simulink library "lib_dGrid"  (R2023b)
settings: Solver=VariableStepAuto  StartTime=0.0  StopTime=10.0  RelTol=1e-3
values from neighbouring files (symbols this model uses):
  C_PM = 10e-3    (= 0.01)    [my_MMC_param.m]
  Cbase = 1/Zbase/wb    (= 3.10849498226e-05)    [my_MMC_param.m]
  f0 = 50/fb    (= 1)    [my_MMC_param.m]
  Fn_filter = 1000    [my_MMC_param.m]
  Fnom = 50    [my_MMC_param.m]
  GFL_APC = 1    [Analysis_Main.m]    (also in initSimu.m; my_MMC_param.m)
  GFL_DVC = 2    [Analysis_Main.m]    (also in initSimu.m; my_MMC_param.m)
  GFM_APC = 3; (values programmed in EMT models)    [Analysis_Main.m]    (also in initSimu.m; my_MMC_param.m = 3)
  GFM_VF = 0    [my_MMC_param.m]
  Ibase = 2*Sbase/(3*Ubase)    [my_MMC_param.m]
  Idcb = Sbase/Udcb    [my_MMC_param.m]
  Ki_Iccsc = 5.15    [my_MMC_param.m]
  Ki_Ireg = CCCTRL.CC.ki    [my_MMC_param.m]
  Ki_Izscc = 100    [my_MMC_param.m]
  Ki_PLL = 1/(CCCTRL.PLL.v0*CCCTRL.PLL.T^2)    [my_MMC_param.m]
  Ki_Preg = 1.0*10    (= 10)    [my_MMC_param.m]
  Ki_Qreg = 1.0*10    (= 10)    [my_MMC_param.m]
  Ki_VAC_GFL = 50    [my_MMC_param.m]
  Ki_VACreg = 10    [my_MMC_param.m]
  Ki_VDCreg = 10    [my_MMC_param.m]
  Ki_WtReg = Kp_WtReg / 0.025    (= 1600)    [my_MMC_param.m]
  Kp_Iccsc = 0.21    [my_MMC_param.m]
  Kp_Ireg = CCCTRL.CC.kp    [my_MMC_param.m]
  Kp_Izscc = 10    [my_MMC_param.m]
  Kp_PLL = 2/CCCTRL.PLL.v0/CCCTRL.PLL.T    [my_MMC_param.m]
  Kp_Preg = 0.5/3*1    (= 0.166666666667)    [my_MMC_param.m]
  Kp_Qreg = 0.5/3*1    (= 0.166666666667)    [my_MMC_param.m]
  Kp_VAC_GFL = 0.5    [my_MMC_param.m]
  Kp_VACreg = 0.01    [my_MMC_param.m]
  Kp_VDCreg = 1    [my_MMC_param.m]
  Kp_WtReg = 40    [my_MMC_param.m]
  Kpv_GFM = 1    [my_MMC_param.m]
  Kpwm = 0.5    [my_MMC_param.m]
  Larm = Larm_pu*(Zbase/wb)    (= 0.0488923985178)    [my_MMC_param.m]
  Lff = Larm_pu/2    (= 0.075)    [my_MMC_param.m]
  Limits_Ireg = [ 2.0  -2.0]    [my_MMC_param.m]
  Limits_Preg = [ 2, -2 ]    [my_MMC_param.m]
  Limits_Qreg = 2*[ 0.42, -0.42 ]    [my_MMC_param.m]
  Limits_VACreg = [ 1.3  -1.3]    [my_MMC_param.m]
  Limits_VDCreg = [ 2.0  -2.0]    [my_MMC_param.m]
  MMC1 = MMC    [Analysis_Main.m]    (also in initSimu.m)
  Nb_PM = 400    [my_MMC_param.m]
  PhaseDelay = 1.0*Ts_Control*2*pi*50    (= 0.0628318530718)    [my_MMC_param.m]
  Pnom = 1000e6    (= 1000000000)    [my_MMC_param.m]
  Rarm = Rarm_pu*Zbase    (= 0.1536)    [my_MMC_param.m]
  Slope_Pref = 0.5    [my_MMC_param.m]
  Slope_Qref = 0.5    [my_MMC_param.m]
  Slope_Vdc_ref = Vnom_dc/2    (= 320000)    [my_MMC_param.m]
  Tdeblock = 1.5    [my_MMC_param.m]
  Ton_CROSSreg = Ton_PQreg+3    (= 7)    [my_MMC_param.m]
  Ton_PQreg = 4    [my_MMC_param.m]
  Ton_VDCreg = 1.5    [my_MMC_param.m]
  Ts = Ts_Control    (= 0.0002)    [my_MMC_param.m]
  Ts_Control = Ts_Power*2    (= 0.0002)    [my_MMC_param.m]
  Ts_Power = 20e-6 * 5    (= 0.0001)    [my_MMC_param.m]
  Ubase = sqrt(2/3)*Vnom_sec    [my_MMC_param.m]
  Udcb = 2*Ubase    [my_MMC_param.m]
  Vc0_PM = 0    [my_MMC_param.m]
  Vnom_dc = 640e3    (= 640000)    [my_MMC_param.m]
  Vnom_sec = 320e3    (= 320000)    [my_MMC_param.m]
  wb = 2*pi*fb    (= 314.159265359)    [my_MMC_param.m]
  Wt_ref_pu = 0.5 * C_PM * (Vnom_dc/Nb_PM)^2 * Nb_PM * 6 / Pnom    (= 0.03072)    [my_MMC_param.m]
undefined symbols (not defined in the file or in its folder): ControlSampleTime, DiscIntNeverNeededParam, MMC, PLL, VSM
libraries: simulink x50, spsCurrentMeasurementLib x20, spsSecondOrderFilterLib x20, spsDiodeLib x12, spsControlledVoltageSourceLib x12, spsSeriesRLCBranchLib x10, spsFirstOrderFilterLib x9, spsVoltageMeasurementLib x8, spsMeanLib x7, FriedrichLibrary x6, $bdroot x6, powerlib_extras x4
(part 3 of 8)

== system lib_dGrid/MMC-configurable control modes/MMC Control/APC & Q//Vac Regulator ==
  note: Reactive Power Regulator
  note: Active Power Regulator
  Pmeas : Inport  PortDimensions=1
  Pref : Inport  Port=2  PortDimensions=1  SampleTime=Ts
  Qmes : Inport  Port=3  PortDimensions=1
  Qref : Inport  Port=4  PortDimensions=1
  VdVq_mes : Inport  Port=5  PortDimensions=2
  Enable : EnablePort  StatesWhenEnabling=reset
  Constant : Constant  Value=Ctrl.IsVacGFL
  Discrete-Time Integrator : DiscreteIntegrator  SampleTime=Ts  LimitOutput=on  UpperSaturationLimit=Limits_Qreg(1)  LowerSaturationLimit=Limits_Qreg(2)  ICPrevOutput=DiscIntNeverNeededParam  ICPrevScaledInput=DiscIntNeverNeededParam
  Discrete-Time Integrator1 : DiscreteIntegrator  SampleTime=Ts  LimitOutput=on  UpperSaturationLimit=Limits_Preg(1)  LowerSaturationLimit=Limits_Preg(2)  ICPrevOutput=DiscIntNeverNeededParam  ICPrevScaledInput=DiscIntNeverNeededParam
  Product{,1..3} (4 alike) : Product  RndMeth=Zero
  Rtot_pu1 : Gain  Gain=-1  SaturateOnIntegerOverflow=on  OutDataTypeStr=Inherit: Same as input  ParamDataTypeStr=Inherit: Same as input
  Saturation1 : Saturate  UpperLimit=Limits_Preg(1)  LowerLimit=Limits_Preg(2)  SampleTime=Ts
  Saturation2 : Saturate  UpperLimit=Limits_Qreg(1)  LowerLimit=Limits_Qreg(2)
  Sum : Sum  Inputs=|-+
  Sum1 : Sum  Inputs=|-+
  Sum2 : Sum  InputSameDT=on  SaturateOnIntegerOverflow=on  SampleTime=Ts  OutDataTypeStr=Inherit: Same as first input
  Sum6 : Sum  InputSameDT=on  SaturateOnIntegerOverflow=on  SampleTime=Ts  OutDataTypeStr=Inherit: Same as first input
  Switch3 : Switch  Criteria=u2 > Threshold  Threshold=0.5  OutDataTypeStr=double  SaturateOnIntegerOverflow=off  InputSameDT=off
  VAC control : Subsystem
  VdcNom_SM : Constant  Value=Kp_Qreg
  VdcNom_SM1 : Constant  Value=Ki_Qreg
  VdcNom_SM2 : Constant  Value=Kp_Preg  SampleTime=Ts
  VdcNom_SM3 : Constant  Value=Ki_Preg  SampleTime=Ts
  Zero-Order Hold : ZeroOrderHold  Commented=through  SampleTime=Ts
  Zero-Order Hold1 : ZeroOrderHold  Commented=through  SampleTime=Ts
  Id_ref_Pctrl : Outport  SampleTime=Ts  VectorParamsAs1DForOutWhenUnconnected=off
  Iq_ref : Outport  Port=2  VectorParamsAs1DForOutWhenUnconnected=off
  wires:
  Saturation2/1 -> Rtot_pu1/1
  Switch3/1 -> Iq_ref/1
  Sum6/1 -> Saturation2/1
  Sum/1 -> Product1/2, Product/2
  Product/1 -> Discrete-Time Integrator/1
  Product1/1 -> Zero-Order Hold/1
  VdcNom_SM/1 -> Product1/1
  VdcNom_SM1/1 -> Product/1
  Discrete-Time Integrator/1 -> Sum6/2
  Zero-Order Hold/1 -> Sum6/1
  Qref/1 -> Sum/2
  Rtot_pu1/1 -> Switch3/3
  Constant/1 -> Switch3/2, VAC control/Enable
  VdVq_mes/1 -> VAC control/1(Vdq_meas)
  VAC control/1(Out1) -> Switch3/1
  VdcNom_SM3/1 -> Product2/1
  Product3/1 -> Zero-Order Hold1/1
  Pmeas/1 -> Sum1/1
  Discrete-Time Integrator1/1 -> Sum2/2
  Zero-Order Hold1/1 -> Sum2/1
  Product2/1 -> Discrete-Time Integrator1/1
  Sum1/1 -> Product3/2, Product2/2
  Pref/1 -> Sum1/2
  Saturation1/1 -> Id_ref_Pctrl/1
  VdcNom_SM2/1 -> Product3/1
  Sum2/1 -> Saturation1/1
  Qmes/1 -> Sum/1

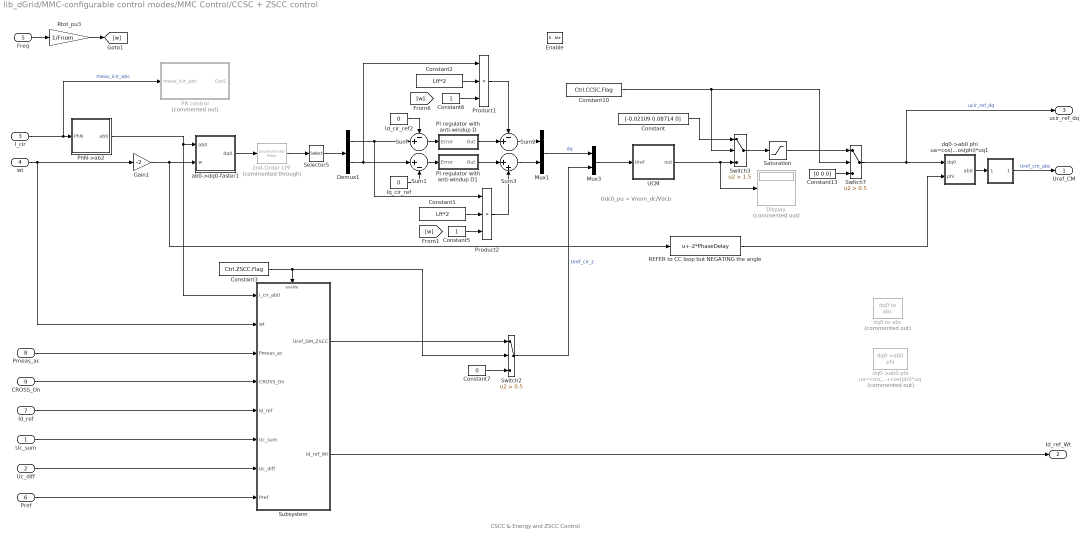
== system lib_dGrid/MMC-configurable control modes/MMC Control/CCSC + ZSCC control ==
  note: CSCC & Energy and ZSCC Control
  note: Udc0_pu = Vnom_dc/Vdcb
  Uc_sum : Inport
  Uc_diff : Inport  Port=2
  I_cir : Inport  Port=3
  wt : Inport  Port=4
  Freq : Inport  Port=5  PortDimensions=1
  Pref : Inport  Port=6  PortDimensions=1
  Id_ref : Inport  Port=7  PortDimensions=1
  Pmeas_ac : Inport  Port=8  PortDimensions=1
  CROSS_On : Inport  Port=9  PortDimensions=1
  Enable : EnablePort  StatesWhenEnabling=reset
  " " : Subsystem
  2nd-Order LPF : spsSecondOrderFilterLib/Second-Order Filter  Commented=through  FilterType=Lowpass  Fo=Fn_filter  Zeta=Zeta_filter  Ts=Ts  Initialize=off  Vac_Init="[0,  0,  60]"  Vdc_Init=0  PlotResponse=off  FreqRange=[0, 500, 1]
      settings: LibrarySourceBlock=|
      | sps_lib/Control/Filters/Second-Order
      | Filter
  Constant : Constant  Value=[-0.02109 0.08714 0]
  Constant1 : Constant  Value=Lff*2  SampleTime=Ts_Control
  Constant10 : Constant  Value=Ctrl.CCSC.Flag
  Constant13 : Constant  Value=[0 0 0]
  Constant2 : Constant  Value=Lff*2  SampleTime=Ts_Control
  Constant3 : Constant  Value=Ctrl.ZSCC.Flag
  Constant5 : Constant
  Constant6 : Constant
  Constant7 : Constant  Value=0
  Demux1 : Demux  Outputs=2
  Display : Display  Commented=on
  Gain1 : Gain  Gain=-2
  Id_cir_ref2 : Constant  Value=0
  Iq_cir_ref : Constant  Value=0
  Mux1 : Mux  Inputs=2
  Mux3 : Mux  Inputs=[2 1]
  PI regulator with anti-windup D : Subsystem  DialogController=POWERSYS.PowerSysDialog  mask(Discrete PI Controller){Kp=Kp_Iccsc, Ki=Ki_Iccsc, Par_Limits=Limits_Ireg, Init=0, Ts=Ts_Control}
      mask prompts: Kp "Proportional gain (Kp):"; Ki "Integral gain (Ki):"; Par_Limits "Output limits: [ Upper   Lower ]"; Init "Output initial value:"; Ts "Sample time:"
      mask help: This block implements a discrete PI controller.
      mask init:
      | UpperLimit=Par_Limits(1);
      | LowerLimit=Par_Limits(2);
      | power_initmask();
      mask Help: This block is part of a subset of blocks in the Extras library that does not have documentation associated with it, other than the block mask description.
      mask Display: disp('PI');
  PI regulator with anti-windup D1 : Subsystem  DialogController=POWERSYS.PowerSysDialog  mask(Discrete PI Controller){Kp=Kp_Iccsc, Ki=Ki_Iccsc, Par_Limits=Limits_Ireg, Init=0, Ts=Ts_Control}
      mask prompts: Kp "Proportional gain (Kp):"; Ki "Integral gain (Ki):"; Par_Limits "Output limits: [ Upper   Lower ]"; Init "Output initial value:"; Ts "Sample time:"
      mask help: This block implements a discrete PI controller.
      mask init:
      | UpperLimit=Par_Limits(1);
      | LowerLimit=Par_Limits(2);
      | power_initmask();
      mask Help: This block is part of a subset of blocks in the Extras library that does not have documentation associated with it, other than the block mask description.
      mask Display: disp('PI');
  PR control : Subsystem  Commented=on
  PhN->ab2 : Subsystem  AncestorBlock=FriedrichLibrary/Transformations/PhN->ab0
      mask Display:
      | plot([0 1], [0,1])
      | plot([0.1 0.25 0.4 0.25 0.25], [0.5 0.6 0.5 0.6 0.8]) % Stern
      | text(0.05,1,'PhN','VerticalAlignment','Top')
      | text(0.55, 0.3,'\alpha\beta0','texmode','on')
  Product1 : Product  Inputs=3  RndMeth=Zero
  Product2 : Product  Inputs=3  RndMeth=Zero
  REFER to CC loop but NEGATING the angle : Bias  Bias=-2*PhaseDelay  SaturateOnIntegerOverflow=off
  Rtot_pu3 : Gain  Gain=1/Fnom  SaturateOnIntegerOverflow=on  OutDataTypeStr=Inherit: Same as input  ParamDataTypeStr=Inherit: Same as input
  Saturation : Saturate  UpperLimit=Limits_Ireg(1)  LowerLimit=Limits_Ireg(2)
  Selector5 : Selector  InputPortWidth=3  IndexOptions=Index vector (dialog)  Indices=[1 2]  OutputSizes=1
  Subsystem : Subsystem
  Sum : Sum  Inputs=-+|
  Sum1 : Sum  Inputs=|+-
  Sum2 : Sum  Inputs=-+|
  Sum3 : Sum  Inputs=|++
  Switch2 : Switch  Criteria=u2 > Threshold  Threshold=0.5  SaturateOnIntegerOverflow=off  InputSameDT=off
  Switch3 : Switch  Criteria=u2 > Threshold  Threshold=1.5  SaturateOnIntegerOverflow=off  InputSameDT=off
  Switch7 : Switch  Criteria=u2 > Threshold  Threshold=0.5  SaturateOnIntegerOverflow=off  InputSameDT=off
  UCM : Subsystem
  ab0->dq0-faster1 : Subsystem  AncestorBlock=FriedrichLibrary/Transformations/ab0->dq0-faster
      mask Display:
      | plot([0 1], [0,1])
      | text(0.05,0.8,'\alpha\beta0','texmode','on')
      | text(1, 0.5,'dq0','HorizontalAlignment','right')
      | text(0.05,0.3,'\phi','texmode','on')
  dq0 to abc : spsdq0toabcLib/dq0 to abc  Commented=on  Alignment=Aligned with phase A axis
  dq0->ab0 phi ua=cos(phi)*ud-sin(phi)*uq ub=-sin(phi)*ud+cos(phi)*uq : FriedrichLibrary/Transformations/dq0->ab0 phi  Commented=on  SystemSampleTime=-1  VariantActivationTime=update diagram  AllowFlexibleInterface=on  Latency=0  AutoFrameSizeCalculation=off
  dq0->ab0 phi ua=cos(phi)*ud-sin(phi)*uq ub=-sin(phi)*ud+cos(phi)*uq1 : Subsystem  AncestorBlock=FriedrichLibrary/Transformations/dq0->ab0 phi
      mask Display:
      | plot([0 1], [0,1])
      | text(0.05,0.8,'dq0','texmode','on')
      | text(1, 0.5,'\alpha\beta0','HorizontalAlignment','right','texmode','on')
      | text(0.05,0.3,'\phi','texmode','on')
  Uref_CM : Outport  VectorParamsAs1DForOutWhenUnconnected=off
  Id_ref_Wt : Outport  Port=2  VectorParamsAs1DForOutWhenUnconnected=off
  ucir_ref_dq : Outport  Port=3  VectorParamsAs1DForOutWhenUnconnected=off
  wires:
  I_cir/1 -> PR control/1(meas_icir_abc), PhN->ab2/1(PhN)  "meas_icir_abc"
  ab0->dq0-faster1/1(dq0) -> 2nd-Order LPF/1
  Gain1/1 -> REFER to CC loop but NEGATING the angle/1, ab0->dq0-faster1/2(w)
  Sum/1 -> PI regulator with anti-windup D/1(Error)
  Selector5/1 -> Demux1/1
  Id_cir_ref2/1 -> Sum/1
  Demux1/1 -> Sum/2, Product2/1
  Sum1/1 -> PI regulator with anti-windup D1/1(Error)
  Iq_cir_ref/1 -> Sum1/2
  Demux1/2 -> Product1/1, Sum1/1
  Constant2/1 -> Product1/2
  Constant6/1 -> Product1/3
  Product1/1 -> Sum2/1
  Sum2/1 -> Mux1/1
  Product2/1 -> Sum3/2
  Constant1/1 -> Product2/2
  Constant5/1 -> Product2/3
  Sum3/1 -> Mux1/2
  Rtot_pu3/1 -> [w]
  Freq/1 -> Rtot_pu3/1
  PI regulator with anti-windup D/1(Out) -> Sum2/2
  PI regulator with anti-windup D1/1(Out) -> Sum3/1
  Switch7/1 -> ucir_ref_dq/1, dq0->ab0 phi ua=cos(phi)*ud-sin(phi)*uq ub=-sin(phi)*ud+cos(phi)*uq1/1(dq0)  "ucir_ref_dq"
  dq0->ab0 phi ua=cos(phi)*ud-sin(phi)*uq ub=-sin(phi)*ud+cos(phi)*uq1/1("ab0 ") -> " "/1(AB0)
  REFER to CC loop but NEGATING the angle/1 -> dq0->ab0 phi ua=cos(phi)*ud-sin(phi)*uq ub=-sin(phi)*ud+cos(phi)*uq1/2(phi)
  Switch2/1 -> Mux3/2  "Uref_cir_z"
  wt/1 -> Subsystem/2(wt), Gain1/1
  2nd-Order LPF/1 -> Selector5/1
  PhN->ab2/1(ab0) -> Subsystem/1(I_cir_ab0), ab0->dq0-faster1/1(ab0)
  Constant/1 -> Switch3/1
  UCM/1(out) -> Display/1, Switch3/3
  Switch3/1 -> Saturation/1
  Constant7/1 -> Switch2/3
  Mux1/1 -> Mux3/1  "dq"
  Pref/1 -> Subsystem/8(Pref)
  Mux3/1 -> UCM/1(Uref)
  Pmeas_ac/1 -> Subsystem/3(Pmeas_ac)
  CROSS_On/1 -> Subsystem/4(CROSS_On)
  Id_ref/1 -> Subsystem/5(Id_ref)
  Subsystem/1(Uref_DM_ZSCC) -> Switch2/1
  Subsystem/2(Id_ref_Wt) -> Id_ref_Wt/1
  Constant3/1 -> Subsystem/Enable, Switch2/2
  Uc_sum/1 -> Subsystem/6(Uc_sum)
  Uc_diff/1 -> Subsystem/7(Uc_diff)
  Constant13/1 -> Switch7/3
  Saturation/1 -> Switch7/1
  Constant10/1 -> Switch3/2, Switch7/2
  " "/1(abc) -> Uref_CM/1  "Uref_cm_abc"

== system lib_dGrid/MMC-configurable control modes/MMC Control/Classic//Cross GFL ->Id* ==
  Id_Wt : Inport
  Cross_On : Inport  Port=2
  Id_P : Inport  Port=3
  PQreg_On : Inport  Port=4
  Id_Udc : Inport  Port=5
  Iq_ref : Inport  Port=6
  Constant1 : Constant  Value=Ctrl.IsCrossGFL
  Divide : Product  Inputs=**
  Mux : Mux  Inputs=2
  Switch4 : Switch  Criteria=u2 ~= 0  Threshold=0.5  OutDataTypeStr=double  SaturateOnIntegerOverflow=off  InputSameDT=off
  Switch5 : Switch  Criteria=u2 > Threshold  Threshold=0.5  SaturateOnIntegerOverflow=off  InputSameDT=off
  Out1 : Outport
  Out2 : Outport  Port=2
  wires:
  Constant1/1 -> Divide/1
  Id_Wt/1 -> Switch5/1
  Switch5/1 -> Mux/1
  Cross_On/1 -> Divide/2
  Id_P/1 -> Switch4/1
  Divide/1 -> Switch5/2
  PQreg_On/1 -> Switch4/2
  Mux/1 -> Out2/1
  Iq_ref/1 -> Mux/2
  Switch4/1 -> Out1/1, Switch5/3
  Id_Udc/1 -> Switch4/3

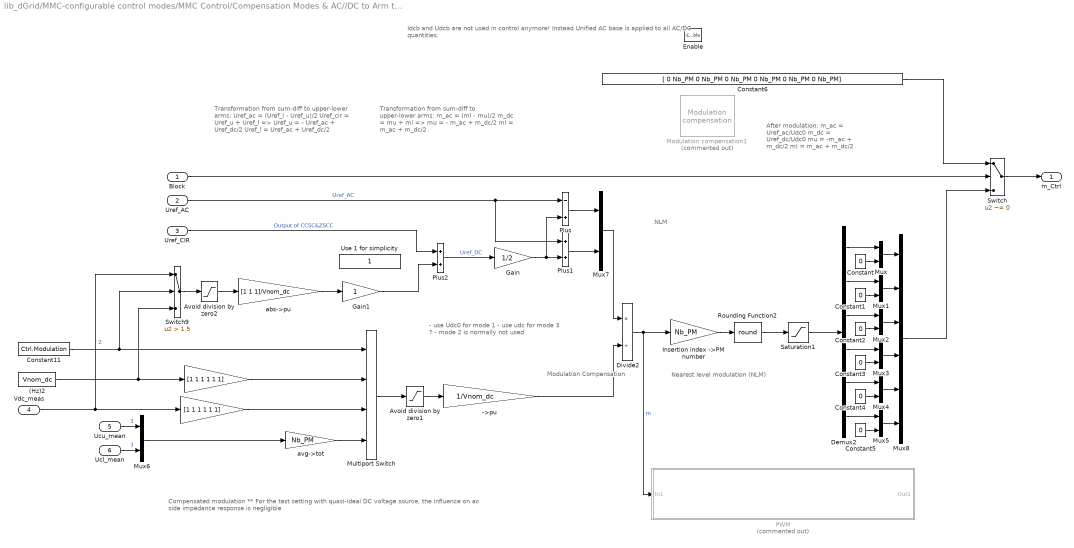
== system lib_dGrid/MMC-configurable control modes/MMC Control/Compensation Modes & AC//DC to Arm transform Number of inserted (Nin) and blocked (Nbl) modules ==
  note: NLM
  note: Modulation
      | Compensation
  note: - use Udc0 for mode 1
      | - use udc for mode 3 ?
      | - mode 2 is normally not used
  note: Transformation from
      | sum-diff to upper-lower arms:
      | m_ac = (ml - mu)/2
      | m_dc = mu + ml =>
      | mu = - m_ac + m_dc/2
      | ml = m_ac + m_dc/2
  note: Idcb and Udcb are not used in control anymore!
      | Instead Unified AC base is applied to all AC/DC quantities.
  note: Compensated modulation
      | ** For the test setting with quasi-ideal DC voltage source, the influence on ac side impedance response is negligible
  note: Transformation from
      | sum-diff to upper-lower arms:
      | Uref_ac = (Uref_l - Uref_u)/2
      | Uref_cir = Uref_u + Uref_l =>
      | Uref_u = - Uref_ac + Uref_dc/2
      | Uref_l = Uref_ac + Uref_dc/2
  note: After modulation:
      | m_ac = Uref_ac/Udc0
      | m_dc = Uref_dc/Udc0
      | mu = -m_ac + m_dc/2
      | ml = m_ac + m_dc/2
  note: Nearest level modulation (NLM)
  Block : Inport
  Uref_AC : Inport  Port=2  PortDimensions=3
  Uref_CIR : Inport  Port=3  PortDimensions=3
  Vdc_meas : Inport  Port=4
  Ucu_mean : Inport  Port=5
  Ucl_mean : Inport  Port=6
  Enable : EnablePort  StatesWhenEnabling=reset
  "  " : Gain  Gain=[1 1 1 1 1 1]
  "     " : Gain  Gain=[1 1 1 1 1 1]
  " (Hz)2" : Constant  Value=Vnom_dc  SampleTime=Ts
  ->pu : Gain  Gain=1/Vnom_dc
  Avoid division by zero1 : Saturate  UpperLimit=Vnom_dc*1.25  LowerLimit=Vnom_dc*0.75
  Avoid division by zero2 : Saturate  UpperLimit=Vnom_dc*1.25  LowerLimit=Vnom_dc*0.75
  Constant{,1..5} (6 alike) : Constant  Value=0
  Constant11 : Constant  Value=Ctrl.Modulation
  Constant6 : Constant  Value=[ 0 Nb_PM 0 Nb_PM 0 Nb_PM 0 Nb_PM 0 Nb_PM 0 Nb_PM]
  Demux2 : Demux  Outputs=6
  Divide2 : Product  Inputs=*/
  Gain : Gain  Gain=1/2
  Gain1 : Gain
  Insertion index ->PM number : Gain  Gain=Nb_PM  SaturateOnIntegerOverflow=on  OutDataTypeStr=Inherit: Same as input  ParamDataTypeStr=Inherit: Same as input
  Modulation compensation1 : $bdroot/MMC/MMC Control/Control output Number of inserted (Nin) and blocked (Nbl) modules/Modulation compensation  Commented=on  SystemSampleTime=-1  SSRTWFcnClass=[]  VariantActivationTime=update diagram  AllowFlexibleInterface=on  Latency=0  AutoFrameSizeCalculation=off
  Multiport Switch : MultiPortSwitch  SaturateOnIntegerOverflow=off
  Mux{,1..7} (8 alike) : Mux  Inputs=2
  Mux8 : Mux  Inputs=6
  PWM : Subsystem  Commented=on
  Plus : Sum  Inputs=-+
  Plus1 : Sum
  Plus2 : Sum
  Rounding Function2 : Rounding  Operator=round
  Saturation1 : Saturate  UpperLimit=Nb_PM  LowerLimit=0
  Switch : Switch  Criteria=u2 ~= 0  SaturateOnIntegerOverflow=off  InputSameDT=off
  Switch9 : Switch  Criteria=u2 > Threshold  Threshold=1.5  OutDataTypeStr=double  SaturateOnIntegerOverflow=off  InputSameDT=off
  Use 1 for simplicity : Constant
  abs->pu : Gain  Gain=[1 1 1]/Vnom_dc
  avg->tot : Gain  Gain=Nb_PM
  m_Ctrl : Outport  VectorParamsAs1DForOutWhenUnconnected=off
  wires:
  Gain/1 -> Plus1/2, Plus/2
  Plus2/1 -> Gain/1  "Uref_DC"
  Uref_AC/1 -> Plus/1, Plus1/1  "Uref_AC"
  abs->pu/1 -> Gain1/1
  Constant11/1 -> Multiport Switch/1, Switch9/2
  Ucu_mean/1 -> Mux6/1  "3"
  " (Hz)2"/1 -> "     "/1, Switch9/3
  Plus/1 -> Mux7/1
  Plus1/1 -> Mux7/2
  Multiport Switch/1 -> Avoid division by zero1/1
  "     "/1 -> Multiport Switch/2
  Switch/1 -> m_Ctrl/1
  Switch9/1 -> Avoid division by zero2/1
  Avoid division by zero2/1 -> abs->pu/1
  Ucl_mean/1 -> Mux6/2  "3"
  Mux6/1 -> avg->tot/1
  avg->tot/1 -> Multiport Switch/4
  Constant6/1 -> Switch/1
  Block/1 -> Switch/2
  "  "/1 -> Multiport Switch/3
  Vdc_meas/1 -> "  "/1, Switch9/1  "2"
  Mux7/1 -> Divide2/1
  ->pu/1 -> Divide2/2
  Avoid division by zero1/1 -> ->pu/1
  Uref_CIR/1 -> Plus2/1  "Output of CCSC&ZSCC"
  Demux2/5 -> Mux4/1
  Rounding Function2/1 -> Saturation1/1
  Mux5/1 -> Mux8/6
  Constant1/1 -> Mux1/2
  Mux4/1 -> Mux8/5
  Mux3/1 -> Mux8/4
  Mux2/1 -> Mux8/3
  Saturation1/1 -> Demux2/1
  Demux2/6 -> Mux5/1
  Demux2/3 -> Mux2/1
  Mux1/1 -> Mux8/2
  Demux2/2 -> Mux1/1
  Demux2/1 -> Mux/1
  Demux2/4 -> Mux3/1
  Constant5/1 -> Mux5/2
  Constant2/1 -> Mux2/2
  Mux/1 -> Mux8/1
  Constant3/1 -> Mux3/2
  Constant4/1 -> Mux4/2
  Insertion index ->PM number/1 -> Rounding Function2/1
  Constant/1 -> Mux/2
  Divide2/1 -> PWM/1(In1), Insertion index ->PM number/1  "m"
  Gain1/1 -> Plus2/2
  Mux8/1 -> Switch/3

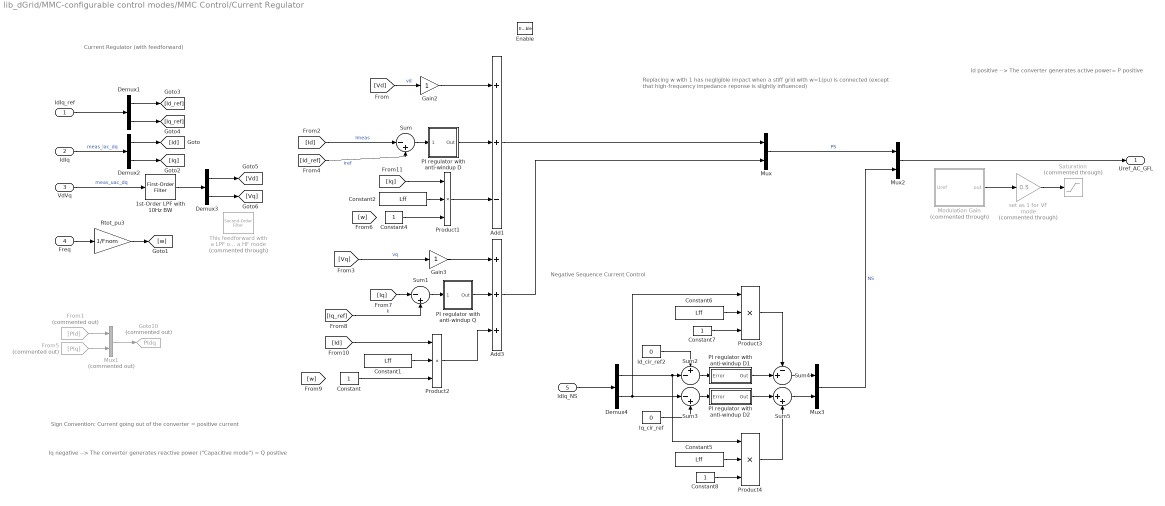
== system lib_dGrid/MMC-configurable control modes/MMC Control/Current Regulator ==
  note: Negative Sequence Current Control
  note: Id positive --> The converter generates active power= P positive
  note: Iq negative --> The converter generates reactive power ("Capacitive mode") = Q positive
  note: Sign Convention: Current going out of the converter = positive current
  note: Current Regulator
      | (with feedforward)
  note: Replacing w with 1 has negligible impact
      | when a stiff grid with w=1(pu) is connected (except that high-frequency impedance reponse is slightly influenced)
  IdIq_ref : Inport  PortDimensions=2
  IdIq : Inport  Port=2  PortDimensions=2
  VdVq : Inport  Port=3  PortDimensions=2
  Freq : Inport  Port=4  PortDimensions=1
  IdIq_NS : Inport  Port=5  PortDimensions=2
  Enable : EnablePort  StatesWhenEnabling=reset
  1st-Order LPF with 10Hz BW : spsFirstOrderFilterLib/First-Order Filter  FilterType=Lowpass  Tc=1/(2*pi*Fn_filter/100)  Ts=Ts  Initialize=off  Vac_Init=[0, 0, 50]  Vdc_Init=0  PlotResponse=off  FreqRange="[0,  200,  1]"
  Add1 : Sum  Inputs=++-
  Add3 : Sum  Inputs=+++
  Constant{,4,7..8} (4 alike) : Constant
  Constant{1..2,5..6} (4 alike) : Constant  Value=Lff  SampleTime=Ts_Control
  Demux{1..4} (4 alike) : Demux  Outputs=2
  From1 : From  Commented=on  GotoTag=PId
  From5 : From  Commented=on  GotoTag=PIq
  Gain2 : Gain
  Gain3 : Gain
  Goto10 : Goto  Commented=on  GotoTag=PIdq  TagVisibility=global
  Id_cir_ref2 : Constant  Value=0
  Iq_cir_ref : Constant  Value=0
  Modulation Gain : Subsystem  Commented=through
  Mux : Mux  Inputs=2
  Mux1 : Mux  Commented=on  Inputs=2
  Mux2 : Mux  Inputs=2
  Mux3 : Mux  Inputs=2
  PI regulator with anti-windup D : Subsystem  DialogController=POWERSYS.PowerSysDialog  mask(Discrete PI Controller){Kp=Kp_Ireg, Ki=Ki_Ireg, Par_Limits=Limits_Ireg, Init=0, Ts=Ts}
      mask prompts: Kp "Proportional gain (Kp):"; Ki "Integral gain (Ki):"; Par_Limits "Output limits: [ Upper   Lower ]"; Init "Output initial value:"; Ts "Sample time:"
      mask help: This block implements a discrete PI controller.
      mask init:
      | UpperLimit=Par_Limits(1);
      | LowerLimit=Par_Limits(2);
      | power_initmask();
      mask Help: This block is part of a subset of blocks in the Extras library that does not have documentation associated with it, other than the block mask description.
      mask Display: disp('PI');
  PI regulator with anti-windup D1 : Subsystem  DialogController=POWERSYS.PowerSysDialog  mask(Discrete PI Controller){Kp=Kp_Ireg/5, Ki=Ki_Ireg/5, Par_Limits=Limits_Ireg/5, Init=0, Ts=Ts}
      mask prompts: Kp "Proportional gain (Kp):"; Ki "Integral gain (Ki):"; Par_Limits "Output limits: [ Upper   Lower ]"; Init "Output initial value:"; Ts "Sample time:"
      mask help: This block implements a discrete PI controller.
      mask init:
      | UpperLimit=Par_Limits(1);
      | LowerLimit=Par_Limits(2);
      | power_initmask();
      mask Help: This block is part of a subset of blocks in the Extras library that does not have documentation associated with it, other than the block mask description.
      mask Display: disp('PI');
  PI regulator with anti-windup D2 : Subsystem  DialogController=POWERSYS.PowerSysDialog  mask(Discrete PI Controller){Kp=Kp_Ireg/5, Ki=Ki_Ireg/5, Par_Limits=Limits_Ireg/5, Init=0, Ts=Ts}
      mask prompts: Kp "Proportional gain (Kp):"; Ki "Integral gain (Ki):"; Par_Limits "Output limits: [ Upper   Lower ]"; Init "Output initial value:"; Ts "Sample time:"
      mask help: This block implements a discrete PI controller.
      mask init:
      | UpperLimit=Par_Limits(1);
      | LowerLimit=Par_Limits(2);
      | power_initmask();
      mask Help: This block is part of a subset of blocks in the Extras library that does not have documentation associated with it, other than the block mask description.
      mask Display: disp('PI');
  PI regulator with anti-windup Q : Subsystem  DialogController=POWERSYS.PowerSysDialog  mask(Discrete PI Controller){Kp=Kp_Ireg, Ki=Ki_Ireg, Par_Limits=Limits_Ireg, Init=0, Ts=Ts}
      mask prompts: Kp "Proportional gain (Kp):"; Ki "Integral gain (Ki):"; Par_Limits "Output limits: [ Upper   Lower ]"; Init "Output initial value:"; Ts "Sample time:"
      mask help: This block implements a discrete PI controller.
      mask init:
      | UpperLimit=Par_Limits(1);
      | LowerLimit=Par_Limits(2);
      | power_initmask();
      mask Help: This block is part of a subset of blocks in the Extras library that does not have documentation associated with it, other than the block mask description.
      mask Display: disp('PI');
  Product{1..4} (4 alike) : Product  Inputs=3  RndMeth=Zero
  Rtot_pu3 : Gain  Gain=1/Fnom  SaturateOnIntegerOverflow=on  OutDataTypeStr=Inherit: Same as input  ParamDataTypeStr=Inherit: Same as input
  Saturation : Saturate  Commented=through  UpperLimit=Limits_Ireg(1)  LowerLimit=Limits_Ireg(2)
  Sum : Sum  Inputs=|-+
  Sum1 : Sum  Inputs=|-+
  Sum2 : Sum  Inputs=+-|
  Sum3 : Sum  Inputs=|-+
  Sum4 : Sum  Inputs=-+|
  Sum5 : Sum  Inputs=|++
  This feedforward with a LPF of 1kHz possibly induce a HF mode : spsSecondOrderFilterLib/Second-Order Filter  Commented=through  FilterType=Lowpass  Fo=Fn_filter  Zeta=Zeta_filter  Ts=Ts  Initialize=off  Vac_Init="[0,  0,  60]"  Vdc_Init=0  PlotResponse=off  FreqRange=[0, 500, 1]
      settings: LibrarySourceBlock=|
      | sps_lib/Control/Filters/Second-Order
      | Filter
  set as 1 for VF mode : Gain  Commented=through  Gain=0.5
  Uref_AC_GFL : Outport  VectorParamsAs1DForOutWhenUnconnected=off
  wires:
  Mux1/1 -> Goto10/1
  PI regulator with anti-windup D/1(Out) -> Add1/2
  PI regulator with anti-windup Q/1(Out) -> Add3/2
  [Vd] -> Gain2/1  "vd"
  Product2/1 -> Add3/3
  [Vq] -> Gain3/1  "vq"
  Demux2/1 -> [Id]
  IdIq/1 -> Demux2/1  "meas_iac_dq"
  [Id] -> Sum/1  "Imeas"
  [Iq] -> Sum1/1
  Demux2/2 -> [Iq]
  From5/1 -> Mux1/2
  From1/1 -> Mux1/1
  Constant4/1 -> Product1/3
  Constant2/1 -> Product1/2
  Constant/1 -> Product2/3
  Constant1/1 -> Product2/2
  Sum1/1 -> PI regulator with anti-windup Q/1(Error)
  Sum/1 -> PI regulator with anti-windup D/1(Error)
  VdVq/1 -> 1st-Order LPF with 10Hz BW/1  "meas_uac_dq"
  Demux3/2 -> [Vq]
  Demux3/1 -> [Vd]
  IdIq_ref/1 -> Demux1/1
  Demux1/2 -> [Iq_ref]
  Demux1/1 -> [Id_ref]
  Rtot_pu3/1 -> [w]
  Freq/1 -> Rtot_pu3/1
  Add1/1 -> Mux/1
  Add3/1 -> Mux/2
  Gain2/1 -> Add1/1
  Gain3/1 -> Add3/1
  set as 1 for VF mode/1 -> Saturation/1
  Modulation Gain/1(out) -> set as 1 for VF mode/1
  [Id] -> Product2/1
  [Iq] -> Product1/1
  Mux/1 -> Mux2/1  "PS"
  1st-Order LPF with 10Hz BW/1 -> Demux3/1
  Sum5/1 -> Mux3/2
  Constant5/1 -> Product4/2
  Demux4/1 -> Product4/1, Sum2/2
  Iq_cir_ref/1 -> Sum3/2
  IdIq_NS/1 -> Demux4/1
  Sum3/1 -> PI regulator with anti-windup D2/1(Error)
  Id_cir_ref2/1 -> Sum2/1
  Sum2/1 -> PI regulator with anti-windup D1/1(Error)
  PI regulator with anti-windup D1/1(Out) -> Sum4/2
  PI regulator with anti-windup D2/1(Out) -> Sum5/1
  Sum4/1 -> Mux3/1
  Product4/1 -> Sum5/2
  Constant7/1 -> Product3/3
  Constant6/1 -> Product3/2
  Demux4/2 -> Product3/1, Sum3/1
  Product3/1 -> Sum4/1
  Constant8/1 -> Product4/3
  Product1/1 -> Add1/3
  [Iq_ref] -> Sum1/2  "k"
  [Id_ref] -> Sum/2  "Iref"
  Mux3/1 -> Mux2/2  "NS"
  Mux2/1 -> Uref_AC_GFL/1

== system lib_dGrid/MMC-configurable control modes/MMC Control/DC Voltage Regulator ** Does current direction influence the +-sign of Id_ref? ==
  note: Taking Vbase as the base voltage for dc voltage
      | Vdc_pu = Vdc_abs / Vbase = Vdc_abs / Vnom_dc * Vnom_dc / Vbase
      | small-signal control loop transfer function is
      | Id_ref = Vdc_abs / Vnom_dc * Hvdc = Vdc_abs / Vnom_dc * Vbase / Vbase * Hvdc = Vdc_pu * Vbase / Vnom_dc * Hvdc
  note: VDC Regulator
  Vdc_meas : Inport  PortDimensions=1
  Vdc_ref : Inport  Port=2  PortDimensions=1
  Enable : EnablePort  StatesWhenEnabling=reset
  "  " : Gain  Gain=-1
  1st-Order HPF : spsFirstOrderFilterLib/First-Order Filter  Commented=through  FilterType=Highpass  Tc=1/(2*pi*20)  Ts=Ts_Control  Initialize=on  Vac_Init=[0, 0, 50]  Vdc_Init=0  PlotResponse=off  FreqRange="[0,  200,  1]"
  2nd-Order LPF : spsSecondOrderFilterLib/Second-Order Filter  Commented=through  FilterType=Lowpass  Fo=Fn_filter/50  Zeta=Zeta_filter  Ts=Ts  Initialize=off  Vac_Init="[0,  0,  60]"  Vdc_Init=0  PlotResponse=off  FreqRange=[0, 500, 1]
      settings: LibrarySourceBlock=|
      | sps_lib/Control/Filters/Second-Order
      | Filter
  Constant : Constant  Commented=on  Value=Vnom_dc*0.9
  Discrete-Time Integrator : DiscreteIntegrator  SampleTime=Ts  LimitOutput=on  UpperSaturationLimit=Limits_VDCreg(1)  LowerSaturationLimit=Limits_VDCreg(2)  ICPrevOutput=DiscIntNeverNeededParam  ICPrevScaledInput=DiscIntNeverNeededParam
  Product : Product  RndMeth=Zero
  Product1 : Product  RndMeth=Zero
  Rtot_pu2 : Gain  Gain=1/Vnom_dc  SaturateOnIntegerOverflow=on  OutDataTypeStr=Inherit: Same as input  ParamDataTypeStr=Inherit: Same as input
  Saturation2 : Saturate  UpperLimit=Limits_VDCreg(1)  LowerLimit=Limits_VDCreg(2)  SampleTime=Ts
  Step : Step  Commented=on  Time=6  SampleTime=0
  Sum : Sum  Inputs=|-+
  Sum6 : Sum  InputSameDT=on  SaturateOnIntegerOverflow=on  SampleTime=Ts  OutDataTypeStr=Inherit: Same as first input
  Switch : Switch  Commented=on  Criteria=u2 > Threshold  SaturateOnIntegerOverflow=off  InputSameDT=off
  VdcNom_SM : Constant  Value=Kp_VDCreg
  VdcNom_SM1 : Constant  Value=Ki_VDCreg
  Zero-Order Hold - Negligible dynamic effect : ZeroOrderHold  Commented=through  SampleTime=Ts
  Id_ref : Outport  VectorParamsAs1DForOutWhenUnconnected=off
  wires:
  Saturation2/1 -> "  "/1
  VdcNom_SM/1 -> Product1/1
  Product/1 -> Discrete-Time Integrator/1
  Product1/1 -> Zero-Order Hold - Negligible dynamic effect/1
  VdcNom_SM1/1 -> Product/1
  Sum6/1 -> Saturation2/1
  Zero-Order Hold - Negligible dynamic effect/1 -> Sum6/1
  Vdc_ref/1 -> Sum/2
  Sum/1 -> Rtot_pu2/1
  Vdc_meas/1 -> 1st-Order HPF/1
  Rtot_pu2/1 -> Product/2, Product1/2
  "  "/1 -> Id_ref/1
  Step/1 -> Switch/2
  Constant/1 -> Switch/1
  Discrete-Time Integrator/1 -> Sum6/2
  1st-Order HPF/1 -> Sum/1

== system lib_dGrid/MMC-configurable control modes/MMC Control/GFL//GFM Switching & Modulation (UCM // DM) & dq0 ->abc ==
  note: VSC CTRL MODE involving current control:
      | >2 for GFM, <0 for VF, otherwise for GFL
  note: proved with negligile effect
  note: Interpretation of Kpwm=0.5 (Method 1): it can be considered to extract a factor of Kpwm from m_ac to get a new modulation factor m_acN, leading to the transformation from sum-diff to upper-lower arms as:
      | m_acN = ml - mu
      | m_dcN = mu + ml =>
      | mu = (-m_acN + m_dc)/2
      | ml = (m_acN + m_dc)/2
  note: The real implementation is:
      | m_ac = (ml - mu)/2
      | m_dc = mu + ml =>
      | mu = - m_ac + m_dc/2
      | ml = m_ac + m_dc/2
  note: Interpretation of Kpwm=0.5 (Method 2): Combining the Kpwm and the neighbored modulation block gives
      | mac_ref = Kpwm*uac_ref / (Udc / Udcb)
      | = Kpwm*uac_ref / (Udc / 2/ Ubase)
      | = (2*Kpwm)*uac_ref / (Udc / Ubase)
      | = uac_ref / (Udc / Ubase)
      | = uac_ref / Udc_pu
      | Compared to TL-VSC with three-phases sharing a same DC voltage, each AC phase of MMC corresponds to one (pair of) summed arm/leg capacitor voltage. In this sense, should AC and DC share a same base voltage?
  note: The DC voltage/capacitor voltage compensation is divided into 2 steps in this model:
      | constant voltage compensation, as applied in this subsystem
      | voltage deviation compensation, as applied in the insersion index generation block
  note: Negative Sequence (NS) Control added on 20-06-2025
      | Fundamental Frequency
  note: Positive Sequence (PS) Control
      | Fundamental Frequency
  Uac_VF : Inport
  Uac_GFM : Inport  Port=2
  Uac_GFL : Inport  Port=3
  ACreg_On : Inport  Port=4
  wt_GFM : Inport  Port=5
  wt_PLL : Inport  Port=6
  wt_VF : Inport  Port=7
  " " : Subsystem
  " 1" : $bdroot/MMC-configurable control modes/MMC Control/GFL//GFM Switching & Modulation (UCM // DM) & dq0 ->abc/   SystemSampleTime=-1  VariantActivationTime=update diagram  AllowFlexibleInterface=on  Latency=0  AutoFrameSizeCalculation=off
  >0 for in1 : Switch  Criteria=u2 > Threshold  SaturateOnIntegerOverflow=off  InputSameDT=off
  >2 for in1 : Switch  Criteria=u2 > Threshold  Threshold=2  SaturateOnIntegerOverflow=off  InputSameDT=off
  Add : Sum
  Constant1 : Constant  Value=CtrlMode
  Constant2 : Constant  Value=0  SampleTime=Ts
  Constant3 : Constant  Value=0  SampleTime=Ts
  Demux : Demux  Outputs=2
  Direct Modulation : $bdroot/MMC-configurable control modes/MMC Control/CCSC + ZSCC control/UCM  SystemSampleTime=-1  VariantActivationTime=update diagram  AllowFlexibleInterface=on  Latency=0  AutoFrameSizeCalculation=off
  Direct Modulation NS : $bdroot/MMC-configurable control modes/MMC Control/CCSC + ZSCC control/UCM  SystemSampleTime=-1  VariantActivationTime=update diagram  AllowFlexibleInterface=on  Latency=0  AutoFrameSizeCalculation=off
  Gain : Gain  Gain=Kpwm
  Gain1 : Gain  Gain=Kpwm
  Gain2 : Gain  Gain=-1
  Mux1 : Mux  Inputs=[2 1]
  Mux2 : Mux  Inputs=[2 1]
  NS-Flag : Gain
  Saturation : Saturate  UpperLimit=Limits_Ireg(1)  LowerLimit=Limits_Ireg(2)
  Saturation1 : Saturate  UpperLimit=Limits_Ireg(1)  LowerLimit=Limits_Ireg(2)
  Switch2 : Switch  Criteria=u2 ~= 0  Threshold=0.5  OutDataTypeStr=double  SaturateOnIntegerOverflow=off  InputSameDT=off
  Switch3 : Switch  Criteria=u2 > Threshold  Threshold=2  SaturateOnIntegerOverflow=off  InputSameDT=off
  dq0 to abc ++ Select Alignment 2 with no phase delay : spsdq0toabcLib/dq0 to abc  Commented=on  Alignment=Aligned with phase A axis
  dq0->ab0 phi ua=cos(phi)*ud-sin(phi)*uq ub=-sin(phi)*ud+cos(phi)*uq : Subsystem  AncestorBlock=FriedrichLibrary/Transformations/dq0->ab0 phi
      mask Display:
      | plot([0 1], [0,1])
      | text(0.05,0.8,'dq0','texmode','on')
      | text(1, 0.5,'\alpha\beta0','HorizontalAlignment','right','texmode','on')
      | text(0.05,0.3,'\phi','texmode','on')
  dq0->ab0 phi ua=cos(phi)*ud-sin(phi)*uq ub=-sin(phi)*ud+cos(phi)*uq1 : $bdroot/MMC-configurable control modes/MMC Control/GFL//GFM Switching & Modulation (UCM // DM) & dq0 ->abc/dq0->ab0 phi ua=cos(phi)*ud-sin(phi)*uq   ub=-sin(phi)*ud+cos(phi)*uq  SystemSampleTime=-1  VariantActivationTime=update diagram  AllowFlexibleInterface=on  Latency=0  AutoFrameSizeCalculation=off
  in2>0 for in1 : Switch  Criteria=u2 > Threshold  SaturateOnIntegerOverflow=off  InputSameDT=off
  refer to TL-VSC control : Bias  Bias=PhaseDelay  SaturateOnIntegerOverflow=off
  ~=0 for in1 : Switch  Criteria=u2 ~= 0  Threshold=0.5  OutDataTypeStr=double  SaturateOnIntegerOverflow=off  InputSameDT=off
  Uref_AC : Outport
  wt : Outport  Port=2
  uac_ref_dq : Outport  Port=3
  wires:
  Demux/1 -> ~=0 for in1/3, >2 for in1/3  "Uac_ref_GFL"
  >2 for in1/1 -> >0 for in1/1
  Uac_GFM/1 -> >2 for in1/1  "Uac_ref_GFM"
  Switch3/1 -> in2>0 for in1/1
  wt_GFM/1 -> Switch3/1  "wt_GFM"
  Constant1/1 -> in2>0 for in1/2, Switch3/2, >2 for in1/2, >0 for in1/2
  ACreg_On/1 -> ~=0 for in1/2, Switch2/2
  wt_PLL/1 -> Switch2/3, Switch3/3  "wt_PLL"
  Uac_VF/1 -> >0 for in1/3  "Uac_ref_VF"
  >0 for in1/1 -> ~=0 for in1/1
  wt_VF/1 -> in2>0 for in1/3  "wt_VF"
  in2>0 for in1/1 -> Switch2/1
  refer to TL-VSC control/1 -> dq0->ab0 phi ua=cos(phi)*ud-sin(phi)*uq ub=-sin(phi)*ud+cos(phi)*uq/2(phi)
  dq0->ab0 phi ua=cos(phi)*ud-sin(phi)*uq ub=-sin(phi)*ud+cos(phi)*uq/1("ab0 ") -> " "/1(AB0)
  Switch2/1 -> refer to TL-VSC control/1, Gain2/1, wt/1  "wt_out"
  Constant3/1 -> Mux2/2
  Saturation/1 -> Mux2/1, uac_ref_dq/1  "uac_ref_dq"
  Mux2/1 -> dq0->ab0 phi ua=cos(phi)*ud-sin(phi)*uq ub=-sin(phi)*ud+cos(phi)*uq/1(dq0)
  " "/1(abc) -> Add/1
  Direct Modulation/1 -> Gain/1
  ~=0 for in1/1 -> Direct Modulation/1  "uac_ref_dq"
  Gain/1 -> Saturation/1
  Uac_GFL/1 -> Demux/1  "Uac_ref_GFL"
  Demux/2 -> Direct Modulation NS/1  "uac_ref_dq_NS"
  Gain1/1 -> Saturation1/1
  Saturation1/1 -> Mux1/1  "uac_ref_dq"
  Mux1/1 -> dq0->ab0 phi ua=cos(phi)*ud-sin(phi)*uq ub=-sin(phi)*ud+cos(phi)*uq1/1
  Direct Modulation NS/1 -> Gain1/1
  dq0->ab0 phi ua=cos(phi)*ud-sin(phi)*uq ub=-sin(phi)*ud+cos(phi)*uq1/1 -> " 1"/1
  Constant2/1 -> Mux1/2
  " 1"/1 -> NS-Flag/1
  Gain2/1 -> dq0->ab0 phi ua=cos(phi)*ud-sin(phi)*uq ub=-sin(phi)*ud+cos(phi)*uq1/2
  Add/1 -> Uref_AC/1
  NS-Flag/1 -> Add/2

== system lib_dGrid/MMC-configurable control modes/MMC Control/PLL, Measurements and Transformation ==
  note: FILTER Setting for Consideration:
      | Only apply LPF to the P&Q measurements of GFL control, not to VSM control scheme (as it is not filter based), and not to the voltage and current measurements of GFL control. The bandwidth can be set as 100 Hz.
      | --- For the LPF-settings with up to 1kHz cutoff frequency, the dynamic effect could be neglected for the 0.1-300 Hz frequency range
  note: Original PQ measurement method
  note: P (pu) = Vd*Id + Vq*Iq
  note: Q (pu) = Vq*Id - Vd*Iq
  note: P positive = Converter generates active power (Inverter Mode)
  note: Q positive = Converter generates reactive power (Capacitive Mode)
  Vabc : Inport  PortDimensions=3
  Iabc : Inport  Port=2  PortDimensions=3
  wt : Inport  Port=3  PortDimensions=1
  2nd-Order LPF 100 Hz : spsSecondOrderFilterLib/Second-Order Filter  FilterType=Lowpass  Fo=Fn_filter/10  Zeta=Zeta_filter  Ts=Ts  Initialize=off  Vac_Init="[0,  0,  60]"  Vdc_Init=0  PlotResponse=off  FreqRange=[0, 500, 1]
      settings: LibrarySourceBlock=|
      | sps_lib/Control/Filters/Second-Order
      | Filter
  "2nd-Order LPF 20Hz -- BETTER NOT USE LPF for VSM synchronization" : spsSecondOrderFilterLib/Second-Order Filter  Commented=through  FilterType=Lowpass  Fo=Fn_filter/50  Zeta=Zeta_filter  Ts=Ts  Initialize=off  Vac_Init="[0,  0,  60]"  Vdc_Init=0  PlotResponse=off  FreqRange=[0, 500, 1]
      settings: LibrarySourceBlock=|
      | sps_lib/Control/Filters/Second-Order
      | Filter
  Add : Sum  Inputs=1
  Demux : Demux  Outputs=2
  Discrete Mean value : powerlib_extras/Discrete Measurements/Discrete  Mean value  Commented=through  Freq=Fnom  Vinit=0  Ts=Ts
  Discrete Mean value1 : powerlib_extras/Discrete Measurements/Discrete  Mean value  Commented=through  Freq=Fnom  Vinit=0  Ts=Ts
  Gain2 : Gain  Gain=-1
  I->pu2 : Gain  Gain=sqrt(3)*Vnom_sec/sqrt(2)/Pnom  SaturateOnIntegerOverflow=on  OutDataTypeStr=Inherit: Same as input  ParamDataTypeStr=Inherit: Same as input
  LPF-5Hz : spsSecondOrderFilterLib/Second-Order Filter  FilterType=Lowpass  Fo=Fn_filter/200  Zeta=Zeta_filter  Ts=Ts  Initialize=off  Vac_Init="[0,  0,  60]"  Vdc_Init=0  PlotResponse=off  FreqRange=[0, 500, 1]
      settings: LibrarySourceBlock=|
      | sps_lib/Control/Filters/Second-Order
      | Filter
  PhN->ab1 : Subsystem  AncestorBlock=FriedrichLibrary/Transformations/PhN->ab0
      mask Display:
      | plot([0 1], [0,1])
      | plot([0.1 0.25 0.4 0.25 0.25], [0.5 0.6 0.5 0.6 0.8]) % Stern
      | text(0.05,1,'PhN','VerticalAlignment','Top')
      | text(0.55, 0.3,'\alpha\beta0','texmode','on')
  PhN->ab2 : Subsystem  AncestorBlock=FriedrichLibrary/Transformations/PhN->ab0
      mask Display:
      | plot([0 1], [0,1])
      | plot([0.1 0.25 0.4 0.25 0.25], [0.5 0.6 0.5 0.6 0.8]) % Stern
      | text(0.05,1,'PhN','VerticalAlignment','Top')
      | text(0.55, 0.3,'\alpha\beta0','texmode','on')
  Product : Product  RndMeth=Zero
  Product1 : Product  RndMeth=Zero
  Second-Order Filter1 : spsSecondOrderFilterLib/Second-Order Filter  Commented=through  FilterType=Lowpass  Fo=Fn_filter  Zeta=Zeta_filter  Ts=Ts  Initialize=off  Vac_Init="[0,  0,  60]"  Vdc_Init=0  PlotResponse=off  FreqRange=[0, 500, 1]
      settings: LibrarySourceBlock=|
      | sps_lib/Control/Filters/Second-Order
      | Filter
  Second-Order Filter2 : spsSecondOrderFilterLib/Second-Order Filter  Commented=through  FilterType=Lowpass  Fo=Fn_filter  Zeta=Zeta_filter  Ts=Ts  Initialize=off  Vac_Init="[0,  0,  60]"  Vdc_Init=0  PlotResponse=off  FreqRange=[0, 500, 1]
      settings: LibrarySourceBlock=|
      | sps_lib/Control/Filters/Second-Order
      | Filter
  Selector1 : Selector  InputPortWidth=3  IndexOptions=Index vector (dialog)  Indices=[1 2]  OutputSizes=1
  Selector2 : Selector  Commented=on  InputPortWidth=3  IndexOptions=Index vector (dialog)  Indices=[1 2]  OutputSizes=1
  Selector3 : Selector  InputPortWidth=2  IndexOptions=Index vector (dialog)  Indices=[2 1]  OutputSizes=1
  Selector4 : Selector  InputPortWidth=3  IndexOptions=Index vector (dialog)  Indices=[1 2]  OutputSizes=1
  Selector5 : Selector  InputPortWidth=3  IndexOptions=Index vector (dialog)  Indices=[1 2]  OutputSizes=1
  Subtract : Sum  Inputs=+-
  Symmetrical PLL : Subsystem  AncestorBlock=FriedrichLibrary/Discrete Stuff/Symmetrical PLL  mask{Kp_PLL=Kp_PLL, Ki_PLL=Ki_PLL, Kd_PLL=0, Ts=Ts_Control}
      mask prompts: Kp_PLL "Proportional Gain PLL"; Ki_PLL "Integral Gain PLL"; Kd_PLL "Differential Gain PLL"; Ts "SampleTime"
      mask DialogControl DescGroupVar Prompt: SRF PLL
      mask DialogControl DescTextVar Prompt: Discrete implementation of a synchronous reference phase locked loop.
  V->pu1 : Gain  Gain=1/(Vnom_sec/sqrt(3)*sqrt(2))  SaturateOnIntegerOverflow=on  OutDataTypeStr=Inherit: Same as input  ParamDataTypeStr=Inherit: Same as input
  ab0->dq0-NS : Subsystem  AncestorBlock=|
      | lib_dGrid/MMC-configurable
      | control modes/MMC Control/PLL, Measurements
      |  and Transformation/ab0->dq0-faster1
      mask Display:
      | plot([0 1], [0,1])
      | text(0.05,0.8,'\alpha\beta0','texmode','on')
      | text(1, 0.5,'dq0','HorizontalAlignment','right')
      | text(0.05,0.3,'\phi','texmode','on')
  ab0->dq0-faster : Subsystem  AncestorBlock=FriedrichLibrary/Transformations/ab0->dq0-faster
      mask Display:
      | plot([0 1], [0,1])
      | text(0.05,0.8,'\alpha\beta0','texmode','on')
      | text(1, 0.5,'dq0','HorizontalAlignment','right')
      | text(0.05,0.3,'\phi','texmode','on')
  ab0->dq0-faster1 : Subsystem  AncestorBlock=FriedrichLibrary/Transformations/ab0->dq0-faster
      mask Display:
      | plot([0 1], [0,1])
      | text(0.05,0.8,'\alpha\beta0','texmode','on')
      | text(1, 0.5,'dq0','HorizontalAlignment','right')
      | text(0.05,0.3,'\phi','texmode','on')
  abc to dq0 : spsabctodq0Lib/abc to dq0  Commented=on  Alignment=Aligned with phase A axis
  from DDSRF-PLL : Subsystem  Commented=on  AncestorBlock=FriedrichLibrary/Transformations/ab0->dq0 PSNS  mask{T1=1/(2*pi*50)}
      mask prompts: T1 "PT1 Settling Time"
      mask Display:
      | plot(0,0,1,1)
      | text(0.05,0.8,'\alpha\beta0','texmode','on')
      | text(1, 0.75,'dq0_PS','HorizontalAlignment','right')
      | text(1, 0.25,'dq0_NS','HorizontalAlignment','right')
      | text(0.05,0.3,'\phi','texmode','on')
  Freq : Outport  VectorParamsAs1DForOutWhenUnconnected=off
  wt_PLL : Outport  Port=2  VectorParamsAs1DForOutWhenUnconnected=off
  VdVq : Outport  Port=3  VectorParamsAs1DForOutWhenUnconnected=off
  IdIq : Outport  Port=4  VectorParamsAs1DForOutWhenUnconnected=off
  P : Outport  Port=5  VectorParamsAs1DForOutWhenUnconnected=off
  Q : Outport  Port=6  VectorParamsAs1DForOutWhenUnconnected=off
  meas_theta_ref : Outport  Port=7  VectorParamsAs1DForOutWhenUnconnected=off
  IdIq_NS : Outport  Port=8  VectorParamsAs1DForOutWhenUnconnected=off
  wires:
  Selector3/1 -> Product1/1
  Selector4/1 -> Product/1, Selector3/1, VdVq/1, Second-Order Filter2/1  "meas_uac_dq"
  Selector5/1 -> IdIq/1, Second-Order Filter1/1, Product1/2, Product/2  "meas_iac_dq"
  Product/1 -> Add/1
  Product1/1 -> Demux/1
  Demux/1 -> Subtract/1
  Demux/2 -> Subtract/2
  Add/1 -> Discrete Mean value/1
  Subtract/1 -> Discrete Mean value1/1
  ab0->dq0-faster/1(dq0) -> Selector4/1
  Vabc/1 -> V->pu1/1
  Iabc/1 -> I->pu2/1
  ab0->dq0-faster1/1(dq0) -> Selector5/1
  Symmetrical PLL/2(phi) -> wt_PLL/1  "wt_PLL"
  Symmetrical PLL/1(f) -> Freq/1  "f"
  PhN->ab1/1(ab0) -> ab0->dq0-faster/1(ab0)
  I->pu2/1 -> PhN->ab2/1(PhN)
  "2nd-Order LPF 20Hz -- BETTER NOT USE LPF for VSM synchronization"/1 -> P/1
  2nd-Order LPF 100 Hz/1 -> Q/1
  wt/1 -> ab0->dq0-faster/2(w), Gain2/1, from DDSRF-PLL/2(w), ab0->dq0-faster1/2(w)  "wt"
  V->pu1/1 -> PhN->ab1/1(PhN), Symmetrical PLL/1(Vabc_PhN)
  Discrete Mean value/1 -> "2nd-Order LPF 20Hz -- BETTER NOT USE LPF for VSM synchronization"/1
  Discrete Mean value1/1 -> 2nd-Order LPF 100 Hz/1
  PhN->ab2/1(ab0) -> ab0->dq0-NS/1(ab0), from DDSRF-PLL/1(ab0), ab0->dq0-faster1/1(ab0)
  Selector1/1 -> LPF-5Hz/1  "meas_iac_dq_NS"
  Symmetrical PLL/3(meas_theta_ref) -> meas_theta_ref/1
  Gain2/1 -> ab0->dq0-NS/2(w)
  ab0->dq0-NS/1(dq0) -> Selector1/1
  from DDSRF-PLL/2(dq0_NS) -> Selector2/1
  Selector2/1 -> ?  "meas_iac_dq_NS"
  LPF-5Hz/1 -> IdIq_NS/1

== system lib_dGrid/MMC-configurable control modes/MMC Control/VF mode ==
  note: AC Voltage Control
  Udq_meas : Inport
  On : Inport  Port=2  PortDimensions=1
  IdIq : Inport  Port=3
  Enable : EnablePort  StatesWhenEnabling=reset
  Add1 : Sum  Commented=on  Inputs=+-
  Constant1 : Constant  Value=50
  Constant2 : Constant  Commented=on  Value=2*pi*f0*50
  Constant9 : Constant  Value=2*pi
  Demux1 : Demux  Outputs=2
  Demux2 : Demux  Outputs=2
  Discrete-Time Integrator : DiscreteIntegrator  InitialCondition=0*pi/180  SampleTime=Ts  ICPrevOutput=DiscIntNeverNeededParam  ICPrevScaledInput=DiscIntNeverNeededParam
  For VF mode : Math  Operator=mod  SignedPower=on
  Gain : Gain  Gain=Lff*0
  Gain1 : Gain  Gain=Lff*0
  Gain2 : Gain  Gain=2*pi
  Integrator (discrete)1 : DiscreteIntegrator  Commented=on  IntegratorMethod=Integration: Backward Euler  gainval=1  SampleTime=Ts_Control  ICPrevOutput=DiscIntNeverNeededParam  ICPrevScaledInput=DiscIntNeverNeededParam
  Mux4 : Mux  Inputs=2
  PI regulator with anti-windup D1 : Subsystem  DialogController=POWERSYS.PowerSysDialog  mask(Discrete PI Controller){Kp=Kp_VACreg, Ki=Ki_VACreg, Par_Limits=Limits_VACreg, Init=0, Ts=Ts}
      mask prompts: Kp "Proportional gain (Kp):"; Ki "Integral gain (Ki):"; Par_Limits "Output limits: [ Upper   Lower ]"; Init "Output initial value:"; Ts "Sample time:"
      mask help: This block implements a discrete PI controller.
      mask init:
      | UpperLimit=Par_Limits(1);
      | LowerLimit=Par_Limits(2);
      | power_initmask();
      mask Help: This block is part of a subset of blocks in the Extras library that does not have documentation associated with it, other than the block mask description.
      mask Display: disp('PI');
  PI regulator with anti-windup D2 : Subsystem  DialogController=POWERSYS.PowerSysDialog  mask(Discrete PI Controller){Kp=Kp_VACreg, Ki=Ki_VACreg, Par_Limits=Limits_VACreg, Init=0, Ts=Ts}
      mask prompts: Kp "Proportional gain (Kp):"; Ki "Integral gain (Ki):"; Par_Limits "Output limits: [ Upper   Lower ]"; Init "Output initial value:"; Ts "Sample time:"
      mask help: This block implements a discrete PI controller.
      mask init:
      | UpperLimit=Par_Limits(1);
      | LowerLimit=Par_Limits(2);
      | power_initmask();
      mask Help: This block is part of a subset of blocks in the Extras library that does not have documentation associated with it, other than the block mask description.
      mask Display: disp('PI');
  Saturation : Saturate  Commented=through  UpperLimit=1.3  LowerLimit=-1.3
  Should be 0 : Display  Commented=on
  Sum4 : Sum  Inputs=+-|
  Sum5 : Sum  Inputs=|-+
  Sum6 : Sum  Inputs=++|
  Sum7 : Sum  Inputs=|+-
  Switch1 : Switch  Criteria=u2 ~= 0  Threshold=0.5  OutDataTypeStr=double  SaturateOnIntegerOverflow=off  InputSameDT=off
  Ud_ref : Constant
  Udq_ref : Constant  Value=[1 0]
  Uq_ref : Constant  Value=0
  Uref_AC : Outport  VectorParamsAs1DForOutWhenUnconnected=off
  wt_VF : Outport  Port=2  VectorParamsAs1DForOutWhenUnconnected=off
  wires:
  Saturation/1 -> Uref_AC/1
  Mux4/1 -> Saturation/1
  For VF mode/1 -> wt_VF/1  "wt"
  Discrete-Time Integrator/1 -> For VF mode/1
  Constant1/1 -> Gain2/1  "f"
  Constant9/1 -> For VF mode/2
  Switch1/1 -> Demux1/1  "Umeas"
  Demux1/2 -> Sum5/1  "Uq_meas"
  Ud_ref/1 -> Sum4/1
  Demux1/1 -> Sum4/2  "Ud_meas"
  Uq_ref/1 -> Sum5/2
  Udq_meas/1 -> Switch1/1
  On/1 -> Switch1/2
  Udq_ref/1 -> Switch1/3  "Uref"
  Gain1/1 -> Sum7/2
  Gain/1 -> Sum6/1
  Sum4/1 -> PI regulator with anti-windup D1/1(Error)
  Sum6/1 -> Mux4/1
  PI regulator with anti-windup D2/1(Out) -> Sum7/1
  Sum7/1 -> Mux4/2
  PI regulator with anti-windup D1/1(Out) -> Sum6/2
  Sum5/1 -> PI regulator with anti-windup D2/1(Error)
  Gain2/1 -> Add1/1, Discrete-Time Integrator/1
  Constant2/1 -> Add1/2
  Add1/1 -> Integrator (discrete)1/1  "d_w"
  Integrator (discrete)1/1 -> Should be 0/1  "meas_theta_VF"
  Demux2/2 -> [Iq]
  IdIq/1 -> Demux2/1  "meas_iac_dq"
  Demux2/1 -> [Id]
  [Iq] -> Gain/1  "Imeas"
  [Id] -> Gain1/1  "Imeas"
